simulink model "bernuliPASHET"  (Simulink 7.9)
settings: Solver=ode45  StartTime=-10.0  StopTime=50.0  RelTol=1e-3
libraries: simulink x1
settings Model: Creator=Mihail  LastModifiedBy=Mihail

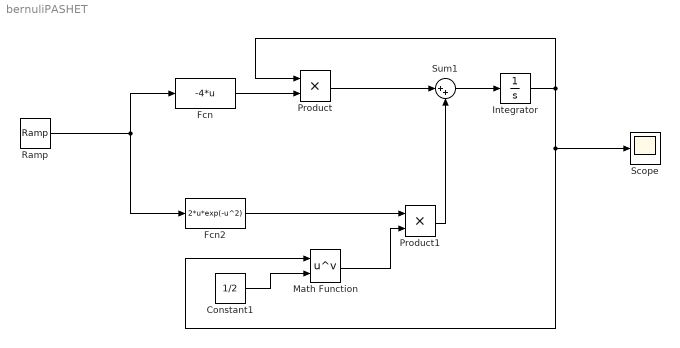
== system bernuliPASHET ==
  Constant1 : Constant  Value=1/2
  Fcn : Fcn  Expr=-4*u
  Fcn2 : Fcn  Expr=2*u*exp(-u^2)
  Integrator : Integrator  InitialCondition=1
  Math Function : Math  Operator=pow  SaturateOnIntegerOverflow=on
  Product : Product  RndMeth=Zero
  Product1 : Product  RndMeth=Zero
  Ramp : simulink/Sources/Ramp  slope=1  start=1  X0=1
  Scope : Scope
  Sum1 : Sum  Inputs=|++
  wires:
  Integrator/1 -> Math Function/1, Product/1, Scope/1
  Fcn2/1 -> Product1/1
  Math Function/1 -> Product1/2
  Product1/1 -> Sum1/2
  Sum1/1 -> Integrator/1
  Ramp/1 -> Fcn/1, Fcn2/1
  Product/1 -> Sum1/1
  Fcn/1 -> Product/2
  Constant1/1 -> Math Function/2
